simulink model "Sim_Forcing_003h_expe_infra5_full_control4"  (Simulink 7.4)
settings: Solver=FixedStepDiscrete  StartTime=0.0  StopTime=inf  FixedStep=0.004  RelTol=1e-3
undefined symbols (not defined in the file or in its folder): DiscIntNeverNeededParam
libraries: simulink x28, gt_rt_lib x22, xpcutilitieslib x4, xpclib x2, dspswit3 x1
(part 4 of 4)

== matlab function Joint Controller (May 7, 2015)1/Inverse Kinematics May 6, 2015/Simplified Inverse Kinematics/Simplified Inverse Kin/Embedded MATLAB Function1 ==
  data: vec input double; out output double
function out = SimpleInvKin( vec )

% We use the NED convention
% This algorithm has a closed form solution and is based on the cosine rule
% However, due to the offset of the centerline of link A4 55 mm below the
% center of rotation of link A3, some small corrections have to be made;
% this is done iteratively by means of a second-order scheme.
% The gist of this routine is to show tha identical results are obtained
% with the fully-fledged 6-DOF inverse algorithm.
%
% The algorithm is also used for computing an initial guess for the
% fully-fledged inverse kinematics algorithm
% The initial guess uses only links A1, A2, A3 and assumes that the
% cabin at the end is straight and level and aligned with the arm
% Thus A4 and A6 are zero and A5 is A2 + A3
%
%   out(7) includes the parameter N
%       N > 0           the number of iterations needed to converge
%       N = -1          the iterative algorithm does not converge
%       N = -2          out of reachable limits
%       N -10<N<-30     upper limit of one of the joints A1-A6 exceeded
%       N -100<N<-110   upper limit of one of the joints A1-A6 exceeded
%
%   Written by Arthur Grunwald, November 11, 2014
%   Added correction because of offset of link A4, Dec 2, 2014
%   Added theta degree-of-freedom April 14, 2015
%   Modified the iterative scheme to second order NR scheme April 24, 2015
%   Modified FAR and CLOSE checks with intersecting circles May 6, 2015

RTD = 180/pi;
DTR = pi/180;

% May 7,2015 soft limits on the links (NED convention)
SL = [   159    129     87      349    60    349
        -159    -19    -87     -349   -60   -349];

% define length of the links

l1          = 50.;   % arm length in cm
l2          = 130.;
l3          = 66.;
l4          = 36.5;
l5          = 29.;
offset      = 5.5;             % vertical offset of the center line of
% joint 4 from centerline of arm A3
% joint 4 from centerline of arm A3
Height_A2   = 104.5 + 106;     % height link A2 above the ground

x = vec(1);
y = vec(2);
z = vec(3);

theta = vec(5);
cos_theta = cos(DTR*vec(5));
sin_theta = sin(DTR*vec(5));

N = 1;
out = zeros(7,1);

% compute dimensions of triangle
l = sqrt(x*x + y*y);
e = l - l1 - l5*cos_theta;
h = -(Height_A2 + z)-l5*sin_theta;
d = sqrt(e^2 + h^2);

% check whether the FAR location of C is reachable
b = l2;
c = l3 + l4;
margin = 5; % margin is 5 cm
if d > b + c - margin
    out(1:6,1) = vec(7:12); % return angles 'as is'
    out(3,1) = -90;
    out(7,1) = -2;
    return
end

% check whether the CLOSE location of C is reachable
if d + c - margin < b
    out(1:6,1) = vec(7:12); % return angles 'as is'
    out(3,1) = -90;
    out(7,1) = -2;
    return
end

% This iterative loop serves to correct for the offset of link A4
% A first good guess is to assume that beta is initially 90 deg
% A second-order scheme is used

A3 = vec(9);
beta = A3 + 180.;

while(1)
    
    sin_beta = sin(beta*DTR);
    sin2_beta = sin_beta*sin_beta;
    cos_beta = cos(beta*DTR);
    
    b = l2 - offset/sin_beta;
    c = l3 + l4 - offset*cos_beta/sin_beta;
    
    db_dbeta = offset * cos_beta/sin2_beta;
    dc_dbeta = offset/sin2_beta;
    
    A = (b*b + c*c - d*d);
    B = (2*b*c);
    dA_dbeta = (2*b*db_dbeta + 2*c*dc_dbeta);
    dB_dbeta = 2*(db_dbeta*c + b*dc_dbeta);
    eps = cos_beta - A/B;
    deps_dbeta = -sin_beta - (dA_dbeta*B - A*dB_dbeta)/B^2;
    dbeta = -RTD*eps/deps_dbeta;
    beta = beta + dbeta;
    
    if abs(dbeta) < 1.e-5
        break
    end
    N = N + 1;
    if N > 100
        N = -2;
        out(1:6,1) = vec(7:12); % return angles 'as is'
        out(3,1) = -90;
        out(7,1) = N;
        break;
    end
end

% employ cosine rule on angles alpha and beta of triangle
cos_alpha = (b*b + d*d - c*c)/(2*b*d);

alpha = RTD*acos(cos_alpha);
delta = RTD*atan2(h, e);

% the link angles
A1 = RTD*atan2(y, x);
A2 = alpha + delta;
A3 = beta - 180;
A4 = 0;
A5 = -(A2 + A3) + theta;
A6 = 0;

J_ANG = [A1 A2 A3 A4 A5 A6]';
out(1:6,1) = J_ANG;

% tests whether the links are within the set soft limits
for i = 1 : 6
    if J_ANG(i) >= SL(1,i)
        N = -10-i;
    elseif J_ANG(i) <= SL(2,i)
        N = -100-i;
    end
end

out(7,1) = N;

end
